simulink model "Projeto_Distribuicao"  (R2018b)
settings: Solver=VariableStepDiscrete  StartTime=0.0  StopTime=2  RelTol=1e-3
libraries: powerlib x50, powerlib_meascontrol x3
settings Model: Creator=ricar  LastModifiedBy=ricar

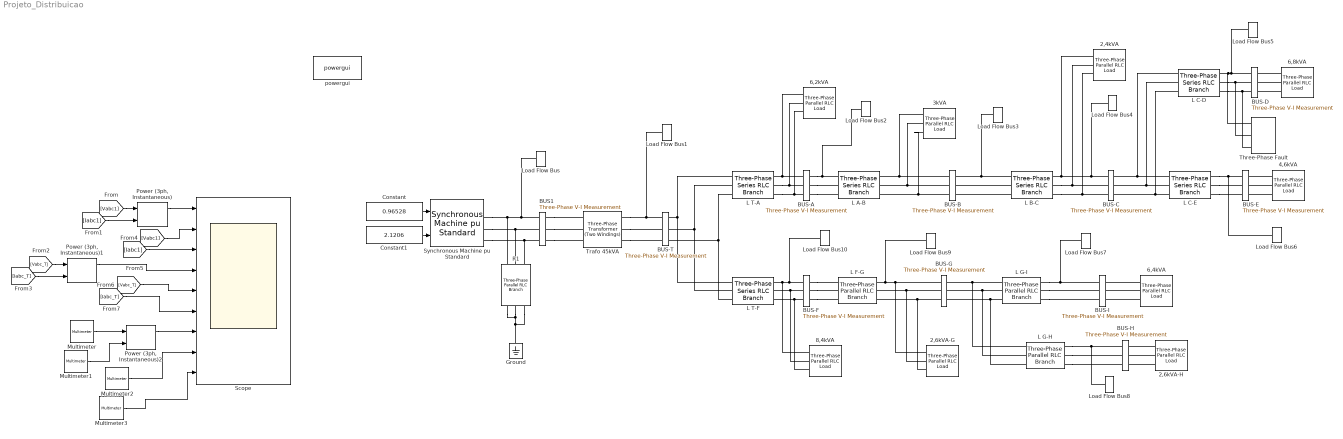
== system Projeto_Distribuicao ==
  2,4kVA : powerlib/Elements/Three-Phase Parallel RLC Load  LConnTagsString=A|B|C  Configuration=Y (grounded)  NominalVoltage=380  Vabc=[1e3 1e3 1e3]  Vabcp=[1e3 1e3 1e3]  NominalFrequency=60  UnbalancedPower=off  ActivePower=2.4e3  InductivePower=0  CapacitivePower=0  Pabc=[10e3 9e3 11e3]  QLabc=[100 90 110]  QCabc=[100 90 110]  Pabcp=[10e3 9e3 11e3]  QLabcp=[100 90 110]  QCabcp=[100 90 110]  Measurements=Branch voltages and currents  LoadType=constant Z
  2,6kVA-G : powerlib/Elements/Three-Phase Parallel RLC Load  LConnTagsString=A|B|C  Configuration=Y (grounded)  NominalVoltage=380  Vabc=[1e3 1e3 1e3]  Vabcp=[1e3 1e3 1e3]  NominalFrequency=60  UnbalancedPower=off  ActivePower=2.6e3  InductivePower=0  CapacitivePower=0  Pabc=[10e3 9e3 11e3]  QLabc=[100 90 110]  QCabc=[100 90 110]  Pabcp=[10e3 9e3 11e3]  QLabcp=[100 90 110]  QCabcp=[100 90 110]  Measurements=Branch voltages and currents  LoadType=constant Z
  2,6kVA-H : powerlib/Elements/Three-Phase Parallel RLC Load  LConnTagsString=A|B|C  Configuration=Y (grounded)  NominalVoltage=380  Vabc=[1e3 1e3 1e3]  Vabcp=[1e3 1e3 1e3]  NominalFrequency=60  UnbalancedPower=off  ActivePower=2.6e3  InductivePower=0  CapacitivePower=0  Pabc=[10e3 9e3 11e3]  QLabc=[100 90 110]  QCabc=[100 90 110]  Pabcp=[10e3 9e3 11e3]  QLabcp=[100 90 110]  QCabcp=[100 90 110]  Measurements=Branch voltages and currents  LoadType=constant Z
  3kVA : powerlib/Elements/Three-Phase Parallel RLC Load  LConnTagsString=A|B|C  Configuration=Y (grounded)  NominalVoltage=380  Vabc=[1e3 1e3 1e3]  Vabcp=[1e3 1e3 1e3]  NominalFrequency=60  UnbalancedPower=off  ActivePower=3e3  InductivePower=0  CapacitivePower=0  Pabc=[10e3 9e3 11e3]  QLabc=[100 90 110]  QCabc=[100 90 110]  Pabcp=[10e3 9e3 11e3]  QLabcp=[100 90 110]  QCabcp=[100 90 110]  Measurements=Branch voltages and currents  LoadType=constant Z
  4,6kVA : powerlib/Elements/Three-Phase Parallel RLC Load  LConnTagsString=A|B|C  Configuration=Y (grounded)  NominalVoltage=380  Vabc=[1e3 1e3 1e3]  Vabcp=[1e3 1e3 1e3]  NominalFrequency=60  UnbalancedPower=off  ActivePower=4.6e3  InductivePower=0  CapacitivePower=0  Pabc=[10e3 9e3 11e3]  QLabc=[100 90 110]  QCabc=[100 90 110]  Pabcp=[10e3 9e3 11e3]  QLabcp=[100 90 110]  QCabcp=[100 90 110]  Measurements=Branch voltages and currents  LoadType=constant Z
  6,2kVA : powerlib/Elements/Three-Phase Parallel RLC Load  LConnTagsString=A|B|C  Configuration=Y (grounded)  NominalVoltage=380  Vabc=[1e3 1e3 1e3]  Vabcp=[1e3 1e3 1e3]  NominalFrequency=60  UnbalancedPower=off  ActivePower=6.2e3  InductivePower=0  CapacitivePower=0  Pabc=[10e3 9e3 11e3]  QLabc=[100 90 110]  QCabc=[100 90 110]  Pabcp=[10e3 9e3 11e3]  QLabcp=[100 90 110]  QCabcp=[100 90 110]  Measurements=Branch voltages and currents  LoadType=constant Z
  6,4kVA : powerlib/Elements/Three-Phase Parallel RLC Load  LConnTagsString=A|B|C  Configuration=Y (grounded)  NominalVoltage=380  Vabc=[1e3 1e3 1e3]  Vabcp=[1e3 1e3 1e3]  NominalFrequency=60  UnbalancedPower=off  ActivePower=6.4e3  InductivePower=0  CapacitivePower=0  Pabc=[10e3 9e3 11e3]  QLabc=[100 90 110]  QCabc=[100 90 110]  Pabcp=[10e3 9e3 11e3]  QLabcp=[100 90 110]  QCabcp=[100 90 110]  Measurements=Branch voltages and currents  LoadType=constant Z
  6,8kVA : powerlib/Elements/Three-Phase Parallel RLC Load  LConnTagsString=A|B|C  Configuration=Y (grounded)  NominalVoltage=380  Vabc=[1e3 1e3 1e3]  Vabcp=[1e3 1e3 1e3]  NominalFrequency=60  UnbalancedPower=off  ActivePower=6.8e3  InductivePower=0  CapacitivePower=0  Pabc=[10e3 9e3 11e3]  QLabc=[100 90 110]  QCabc=[100 90 110]  Pabcp=[10e3 9e3 11e3]  QLabcp=[100 90 110]  QCabcp=[100 90 110]  Measurements=Branch voltages and currents  LoadType=constant Z
  8,4kVA : powerlib/Elements/Three-Phase Parallel RLC Load  LConnTagsString=A|B|C  Configuration=Y (grounded)  NominalVoltage=380  Vabc=[1e3 1e3 1e3]  Vabcp=[1e3 1e3 1e3]  NominalFrequency=60  UnbalancedPower=off  ActivePower=8.4e3  InductivePower=0  CapacitivePower=0  Pabc=[10e3 9e3 11e3]  QLabc=[100 90 110]  QCabc=[100 90 110]  Pabcp=[10e3 9e3 11e3]  QLabcp=[100 90 110]  QCabcp=[100 90 110]  Measurements=Branch voltages and currents  LoadType=constant Z
  BUS-A : powerlib/Measurements/Three-Phase V-I Measurement  VoltageMeasurement=phase-to-ground  SetLabelV=on  LabelV=Vabc_A  Vpu=off  VpuLL=off  CurrentMeasurement=yes  SetLabelI=on  LabelI=Iabc_A  Ipu=off  Pbase=100e6  Vbase=500e3  OutputType=Complex  PhasorSimulation=off  PSBequivalent=0
  BUS-B : powerlib/Measurements/Three-Phase V-I Measurement  VoltageMeasurement=phase-to-ground  SetLabelV=on  LabelV=Vabc_B  Vpu=off  VpuLL=off  CurrentMeasurement=yes  SetLabelI=on  LabelI=Iabc_B  Ipu=off  Pbase=100e6  Vbase=500e3  OutputType=Complex  PhasorSimulation=off  PSBequivalent=0
  BUS-C : powerlib/Measurements/Three-Phase V-I Measurement  VoltageMeasurement=phase-to-ground  SetLabelV=on  LabelV=Vabc_C  Vpu=off  VpuLL=off  CurrentMeasurement=yes  SetLabelI=on  LabelI=Iabc_C  Ipu=off  Pbase=100e6  Vbase=500e3  OutputType=Complex  PhasorSimulation=off  PSBequivalent=0
  BUS-D : powerlib/Measurements/Three-Phase V-I Measurement  VoltageMeasurement=phase-to-ground  SetLabelV=on  LabelV=Vabc_D  Vpu=off  VpuLL=off  CurrentMeasurement=yes  SetLabelI=on  LabelI=Iabc_D  Ipu=off  Pbase=100e6  Vbase=500e3  OutputType=Complex  PhasorSimulation=off  PSBequivalent=0
  BUS-E : powerlib/Measurements/Three-Phase V-I Measurement  VoltageMeasurement=phase-to-ground  SetLabelV=on  LabelV=Vabc_E  Vpu=off  VpuLL=off  CurrentMeasurement=yes  SetLabelI=on  LabelI=Iabc_E  Ipu=off  Pbase=100e6  Vbase=500e3  OutputType=Complex  PhasorSimulation=off  PSBequivalent=0
  BUS-F : powerlib/Measurements/Three-Phase V-I Measurement  VoltageMeasurement=phase-to-ground  SetLabelV=on  LabelV=Vabc_F  Vpu=off  VpuLL=off  CurrentMeasurement=yes  SetLabelI=on  LabelI=Iabc_F  Ipu=off  Pbase=100e6  Vbase=500e3  OutputType=Complex  PhasorSimulation=off  PSBequivalent=0
  BUS-G : powerlib/Measurements/Three-Phase V-I Measurement  VoltageMeasurement=phase-to-ground  SetLabelV=on  LabelV=Vabc_G  Vpu=off  VpuLL=off  CurrentMeasurement=yes  SetLabelI=on  LabelI=Iabc_G  Ipu=off  Pbase=100e6  Vbase=500e3  OutputType=Complex  PhasorSimulation=off  PSBequivalent=0
  BUS-H : powerlib/Measurements/Three-Phase V-I Measurement  VoltageMeasurement=phase-to-ground  SetLabelV=on  LabelV=Vabc_H  Vpu=off  VpuLL=off  CurrentMeasurement=yes  SetLabelI=on  LabelI=Iabc_H  Ipu=off  Pbase=100e6  Vbase=500e3  OutputType=Complex  PhasorSimulation=off  PSBequivalent=0
  BUS-I : powerlib/Measurements/Three-Phase V-I Measurement  VoltageMeasurement=phase-to-ground  SetLabelV=on  LabelV=Vabc_I  Vpu=off  VpuLL=off  CurrentMeasurement=yes  SetLabelI=on  LabelI=Iabc_I  Ipu=off  Pbase=100e6  Vbase=500e3  OutputType=Complex  PhasorSimulation=off  PSBequivalent=0
  BUS-T : powerlib/Measurements/Three-Phase V-I Measurement  VoltageMeasurement=phase-to-ground  SetLabelV=on  LabelV=Vabc_T  Vpu=off  VpuLL=off  CurrentMeasurement=yes  SetLabelI=on  LabelI=Iabc_T  Ipu=off  Pbase=100e6  Vbase=500e3  OutputType=Complex  PhasorSimulation=off  PSBequivalent=0
  BUS1 : powerlib/Measurements/Three-Phase V-I Measurement  VoltageMeasurement=phase-to-ground  SetLabelV=on  LabelV=Vabc1  Vpu=off  VpuLL=off  CurrentMeasurement=yes  SetLabelI=on  LabelI=Iabc1  Ipu=off  Pbase=100e6  Vbase=500e3  OutputType=Complex  PhasorSimulation=off  PSBequivalent=0
  Constant : Constant  Value=0.96528
  Constant1 : Constant  Value=2.1206
  Ground : powerlib/Elements/Ground  LConnTagsString=a
  L A-B : powerlib/Elements/Three-Phase Series RLC Branch  LConnTagsString=A|B|C  RConnTagsString=A|B|C  BranchType=R  Resistance=0.032585  Inductance=1e-3  Capacitance=1e-6  Measurements=None
  L B-C : powerlib/Elements/Three-Phase Series RLC Branch  LConnTagsString=A|B|C  RConnTagsString=A|B|C  BranchType=R  Resistance=0.0300125  Inductance=1e-3  Capacitance=1e-6  Measurements=None
  L C-D : powerlib/Elements/Three-Phase Series RLC Branch  LConnTagsString=A|B|C  RConnTagsString=A|B|C  BranchType=R  Resistance=0.0343  Inductance=1e-3  Capacitance=1e-6  Measurements=None
  L C-E : powerlib/Elements/Three-Phase Series RLC Branch  LConnTagsString=A|B|C  RConnTagsString=A|B|C  BranchType=R  Resistance=0.0343  Inductance=1e-3  Capacitance=1e-6  Measurements=None
  L F-G : powerlib/Elements/Three-Phase Parallel RLC Branch  LConnTagsString=A|B|C  RConnTagsString=A|B|C  BranchType=R  Resistance=0.0188531  Inductance=0  Capacitance=0  Measurements=None
      settings: SourceProductName=Simscape Power Systems  SourceProductBaseCode=PS
  L G-H : powerlib/Elements/Three-Phase Parallel RLC Branch  LConnTagsString=A|B|C  RConnTagsString=A|B|C  BranchType=R  Resistance=0.042875  Inductance=0  Capacitance=0  Measurements=None
      settings: SourceProductName=Simscape Power Systems  SourceProductBaseCode=PS
  L G-I : powerlib/Elements/Three-Phase Parallel RLC Branch  LConnTagsString=A|B|C  RConnTagsString=A|B|C  BranchType=R  Resistance=0.0300125  Inductance=0  Capacitance=0  Measurements=None
      settings: SourceProductName=Simscape Power Systems  SourceProductBaseCode=PS
  L T-A : powerlib/Elements/Three-Phase Series RLC Branch  LConnTagsString=A|B|C  RConnTagsString=A|B|C  BranchType=R  Resistance=0.0107732  Inductance=1e-3  Capacitance=1e-6  Measurements=None
  L T-F : powerlib/Elements/Three-Phase Series RLC Branch  LConnTagsString=A|B|C  RConnTagsString=A|B|C  BranchType=R  Resistance=0.0134665  Inductance=1e-3  Capacitance=1e-6  Measurements=None
  Load Flow Bus : powerlib/Measurements/Load Flow Bus  LConnTagsString=a  Phases=single  Connectors=on one side  ID=BUS_1  Vbase=13.8e3  Vref=1  Vangle=0  VLF=1  VLFb=1  VLFc=1  angleLF=0  angleLFb=0  angleLFc=0
      settings: SourceProductName=Simscape Power Systems
  Load Flow Bus1 : powerlib/Measurements/Load Flow Bus  LConnTagsString=a  Phases=single  Connectors=on one side  ID=BUS_T  Vbase=380  Vref=1  Vangle=0  VLF=0.9848  VLFb=1  VLFc=1  angleLF=-8.624  angleLFb=0  angleLFc=0
      settings: SourceProductName=Simscape Power Systems
  Load Flow Bus10 : powerlib/Measurements/Load Flow Bus  LConnTagsString=a  Phases=single  Connectors=on one side  ID=BUS_F  Vbase=380  Vref=1  Vangle=0  VLF=0.983  VLFb=1  VLFc=1  angleLF=-8.624  angleLFb=0  angleLFc=0
      settings: SourceProductName=Simscape Power Systems
  Load Flow Bus2 : powerlib/Measurements/Load Flow Bus  LConnTagsString=a  Phases=single  Connectors=on one side  ID=BUS_A  Vbase=380  Vref=1  Vangle=0  VLF=0.9831  VLFb=1  VLFc=1  angleLF=-8.624  angleLFb=0  angleLFc=0
      settings: SourceProductName=Simscape Power Systems
  Load Flow Bus3 : powerlib/Measurements/Load Flow Bus  LConnTagsString=a  Phases=single  Connectors=on one side  ID=BUS_B  Vbase=380  Vref=1  Vangle=0  VLF=0.9794  VLFb=1  VLFc=1  angleLF=-8.624  angleLFb=0  angleLFc=0
      settings: SourceProductName=Simscape Power Systems
  Load Flow Bus4 : powerlib/Measurements/Load Flow Bus  LConnTagsString=a  Phases=single  Connectors=on one side  ID=BUS_C  Vbase=380  Vref=1  Vangle=0  VLF=0.9766  VLFb=1  VLFc=1  angleLF=-8.624  angleLFb=0  angleLFc=0
      settings: SourceProductName=Simscape Power Systems
  Load Flow Bus5 : powerlib/Measurements/Load Flow Bus  LConnTagsString=a  Phases=single  Connectors=on one side  ID=BUS_D  Vbase=380  Vref=1  Vangle=0  VLF=0.975  VLFb=1  VLFc=1  angleLF=-8.624  angleLFb=0  angleLFc=0
      settings: SourceProductName=Simscape Power Systems
  Load Flow Bus6 : powerlib/Measurements/Load Flow Bus  LConnTagsString=a  Phases=single  Connectors=on one side  ID=BUS_E  Vbase=380  Vref=1  Vangle=0  VLF=0.9756  VLFb=1  VLFc=1  angleLF=-8.624  angleLFb=0  angleLFc=0
      settings: SourceProductName=Simscape Power Systems
  Load Flow Bus7 : powerlib/Measurements/Load Flow Bus  LConnTagsString=a  Phases=single  Connectors=on one side  ID=BUS_I  Vbase=380  Vref=1  Vangle=0  VLF=0.9802  VLFb=1  VLFc=1  angleLF=-8.624  angleLFb=0  angleLFc=0
      settings: SourceProductName=Simscape Power Systems
  Load Flow Bus8 : powerlib/Measurements/Load Flow Bus  LConnTagsString=a  Phases=single  Connectors=on one side  ID=BUS_H  Vbase=380  Vref=1  Vangle=0  VLF=0.9807  VLFb=1  VLFc=1  angleLF=-8.624  angleLFb=0  angleLFc=0
      settings: SourceProductName=Simscape Power Systems
  Load Flow Bus9 : powerlib/Measurements/Load Flow Bus  LConnTagsString=a  Phases=single  Connectors=on one side  ID=BUS_G  Vbase=380  Vref=1  Vangle=0  VLF=0.9815  VLFb=1  VLFc=1  angleLF=-8.624  angleLFb=0  angleLFc=0
      settings: SourceProductName=Simscape Power Systems
  Multimeter : powerlib/Measurements/Multimeter  PhasorSimulation=off  OutputType=Complex  sel=[22 23 24]  L=54  Gain=[1 1 1]  yselected={'Uag: 6,8kVA','Ubg: 6,8kVA','Ucg: 6,8kVA'};  PSBOutputType=1  PSBequivalent=0  AxesSetting=[0,0.1,-100,100]  Display=0  SavedBlockNames=-11
  Multimeter1 : powerlib/Measurements/Multimeter  PhasorSimulation=off  OutputType=Complex  sel=[49 50 51]  L=54  Gain=[1 1 1]  yselected={'Iag: 6,8kVA','Ibg: 6,8kVA','Icg: 6,8kVA'};  PSBOutputType=1  PSBequivalent=0  AxesSetting=[0,0.1,-100,100]  Display=0  SavedBlockNames=-11
  Multimeter2 : powerlib/Measurements/Multimeter  PhasorSimulation=off  OutputType=Complex  sel=[22 23 24]  L=54  Gain=[1 1 1]  yselected={'Uag: 6,8kVA','Ubg: 6,8kVA','Ucg: 6,8kVA'};  PSBOutputType=1  PSBequivalent=0  AxesSetting=[0,0.1,-100,100]  Display=0  SavedBlockNames=-11
  Multimeter3 : powerlib/Measurements/Multimeter  PhasorSimulation=off  OutputType=Complex  sel=[49 50 51]  L=54  Gain=[1 1 1]  yselected={'Iag: 6,8kVA','Ibg: 6,8kVA','Icg: 6,8kVA'};  PSBOutputType=1  PSBequivalent=0  AxesSetting=[0,0.1,-100,100]  Display=0  SavedBlockNames=-11
  "Power (3ph, Instantaneous)" : powerlib_meascontrol/Measurements/Power (3ph, Instantaneous)
      settings: SourceProductName=Simscape Power Systems
  "Power (3ph, Instantaneous)1" : powerlib_meascontrol/Measurements/Power (3ph, Instantaneous)
      settings: SourceProductName=Simscape Power Systems
  "Power (3ph, Instantaneous)2" : powerlib_meascontrol/Measurements/Power (3ph, Instantaneous)
      settings: SourceProductName=Simscape Power Systems
  R1 : powerlib/Elements/Three-Phase Parallel RLC Branch  LConnTagsString=A|B|C  RConnTagsString=A|B|C  BranchType=R  Resistance=1e+6  Inductance=1e-3  Capacitance=1e-6  Measurements=None
      settings: SourceProductName=Simscape Power Systems  SourceProductBaseCode=PS
  Scope : Scope  NumInputPorts=9
  Synchronous Machine pu Standard : powerlib/Machines/Synchronous Machine pu Standard  PresetModel=No  MechanicalLoad=Mechanical power Pm  ShowDetailedParameters=on  RotorType=Round  Units=per unit standard parameters  MeasurementBus=off  NominalParameters=[45e+03 13800 60]  Reactances1=[ 1.81, 0.3, 0.23, 1.76, 0.65, 0.25, 0.15 ]  Reactances2=[2.24 0.17 0.12 1.02 0.13 0.08]  dAxisTimeConstants=Short-circuit  qAxisTimeConstants=Short-circuit  TimeConstants1="[ 4.4849  0.0681  0.1  ]"  TimeConstants2=[ 8.0, 0.03, 1.0, 0.07 ]  TimeConstants3="[  4.49  0.0681  0.0513  ]"  TimeConstants4=[ 8.0, 0.03, 0.3371, 0.0295 ]  TimeConstants5=[ 1.01, 0.053, 0.1 ]  TimeConstants6=[ 1.3201, 0.023, 1.0, 0.07 ]  TimeConstants7=[0.012 0.003 0.003]  TimeConstants8=[ 1.3201, 0.0231, 0.3371, 0.0295 ]  StatorResistance=0.037875  Mechanical=[0.1028 0.02056 2]  PolePairs=20  InitialConditions=[0 -38.2008 0.942468 0.942468 0.942468 -8.69634 -128.696 111.304 2.12064]  SetSaturation=off  Saturation=[0.6404,0.7127,0.8441,0.9214,0.9956,1.082,1.19,1.316,1.457;0.7,0.7698,0.8872,0.9466,0.9969,1.046,1.1,1.151,1.201]  LoadFlowParameters=[1,0,0,0,0]  TsPowergui=0  TsBlock=-1  IterativeModel=Trapezoidal non iterative  IterativeDiscreteModel=Trapezoidal non iterative  BusType=swing  Pref=0  Qref=0  Qmin=-inf  Qmax=inf  PLF=0  QLF=0
      settings: SourceProductName=Simscape Power Systems
  Three-Phase Fault : powerlib/Elements/Three-Phase Fault  InitialStates=0  FaultA=on  FaultB=off  FaultC=off  GroundFault=on  SwitchTimes="[0.2  0.5]"  External=off  SwitchStatus=NaN  FaultResistance=0.001  GroundResistance=0.01  SnubberResistance=1e6  SnubberCapacitance=inf  Measurements=None
  Trafo 45kVA : powerlib/Elements/Three-Phase Transformer (Two Windings)  Winding1Connection=Yg  Winding2Connection=Yg  CoreType=Three single-phase transformers  SetSaturation=off  Hysteresis=off  DataFile='hysteresis'  SetInitialFlux=off  Measurements=None  UNITS=pu  NominalPower=[ 45e3 , 60 ]  Winding1=[ 13.8e3 , 0.002 , 0.08 ]  Winding2=[ 380 , 0.002 , 0.08 ]  Rm=500  Lm=500  L0=0.5  Saturation=[ 0,0 ; 0.0024,1.2 ; 1.0,1.52 ]  InitialFluxes=[ 0.8 , -0.8 , 0.7 ]  MoreParameters=off  BreakLoop=off  DataType=off  TransfoNumber=1
  powergui : powerlib/powergui  Priority=1  SimulationMode=Discrete  SampleTime=50e-6  frequency=60  Iterations=1000  frequencyindice=60  Pbase=100e3  ErrMax=0.0001  UnitsV=V  UnitsW=kW  buscounter=0  FunctionMessages=off  echomessages=off  EnableUseOfTLC=off  CurrentSourceSwitches=off  DisableSnubberDevices=off  DisableRonSwitches=off  DisableVfSwitches=off  DisplayEquations=off  SolverType=Tustin/Backward Euler (TBE)  Interpol=off  ExternalGateDelay=off  methode=off  Ts=100  x0status=blocks  SPID=on  SwTol=0  HookPort=off  RestoreLinks=warning  ResistiveCurrentMeasurement=off  Frange=[0:2:500]  Ylog=off  Xlog=on  ShowGrid=off  save=off  variable=ZData  structure=0  ZoomFFT=off  StartTime=0.0  cycles=1  DisplayStyle=1  fundamental=60  FreqAxis=off  MaxFrequency=1000  frequencyindicesteady=1  RmsSteady=1  display=off
  wires:
  Constant/1 -> Synchronous Machine pu Standard/1
  Constant1/1 -> Synchronous Machine pu Standard/2
  [Iabc1] -> "Power (3ph, Instantaneous)"/2
  [Vabc1] -> "Power (3ph, Instantaneous)"/1
  "Power (3ph, Instantaneous)"/1 -> Scope/1
  [Iabc_T] -> "Power (3ph, Instantaneous)1"/2
  [Vabc_T] -> "Power (3ph, Instantaneous)1"/1
  Multimeter/1 -> "Power (3ph, Instantaneous)2"/1
  Multimeter1/1 -> "Power (3ph, Instantaneous)2"/2
  "Power (3ph, Instantaneous)1"/1 -> Scope/4
  "Power (3ph, Instantaneous)2"/1 -> Scope/7
  [Vabc1] -> Scope/2
  [Iabc1] -> Scope/3
  [Vabc_T] -> Scope/5
  [Iabc_T] -> Scope/6
  Multimeter2/1 -> Scope/8
  Multimeter3/1 -> Scope/9
  connections:
  R1/LConn1 -- Synchronous Machine pu Standard/RConn1 -- Load Flow Bus/LConn1 -- BUS1/LConn1
  R1/LConn2 -- Synchronous Machine pu Standard/RConn2 -- BUS1/LConn2
  R1/LConn3 -- Synchronous Machine pu Standard/RConn3 -- BUS1/LConn3
  BUS1/RConn1 -- Trafo 45kVA/LConn1
  BUS1/RConn2 -- Trafo 45kVA/LConn2
  BUS1/RConn3 -- Trafo 45kVA/LConn3
  Trafo 45kVA/RConn1 -- Load Flow Bus1/LConn1 -- BUS-T/LConn1
  Trafo 45kVA/RConn2 -- BUS-T/LConn2
  Trafo 45kVA/RConn3 -- BUS-T/LConn3
  BUS-T/RConn1 -- L T-F/LConn1 -- L T-A/LConn1
  BUS-T/RConn2 -- L T-F/LConn2 -- L T-A/LConn2
  BUS-T/RConn3 -- L T-F/LConn3 -- L T-A/LConn3
  L T-A/RConn1 -- 6,2kVA/LConn1 -- BUS-A/LConn1
  L T-A/RConn2 -- 6,2kVA/LConn2 -- BUS-A/LConn2
  L T-A/RConn3 -- 6,2kVA/LConn3 -- BUS-A/LConn3
  BUS-A/RConn1 -- Load Flow Bus2/LConn1 -- L A-B/LConn1
  BUS-A/RConn2 -- L A-B/LConn2
  BUS-A/RConn3 -- L A-B/LConn3
  L T-F/RConn1 -- 8,4kVA/LConn1 -- Load Flow Bus10/LConn1 -- BUS-F/LConn1
  L T-F/RConn2 -- 8,4kVA/LConn2 -- BUS-F/LConn2
  L T-F/RConn3 -- 8,4kVA/LConn3 -- BUS-F/LConn3
  BUS-F/RConn1 -- L F-G/LConn1
  BUS-F/RConn2 -- L F-G/LConn2
  BUS-F/RConn3 -- L F-G/LConn3
  BUS-B/LConn1 -- 3kVA/LConn1 -- L A-B/RConn1
  BUS-B/LConn2 -- 3kVA/LConn2 -- L A-B/RConn2
  BUS-B/LConn3 -- 3kVA/LConn3 -- L A-B/RConn3
  BUS-G/LConn1 -- 2,6kVA-G/LConn1 -- Load Flow Bus9/LConn1 -- L F-G/RConn1
  BUS-G/LConn2 -- 2,6kVA-G/LConn2 -- L F-G/RConn2
  BUS-G/LConn3 -- 2,6kVA-G/LConn3 -- L F-G/RConn3
  L B-C/LConn3 -- BUS-B/RConn3
  L B-C/LConn2 -- BUS-B/RConn2
  L B-C/LConn1 -- Load Flow Bus3/LConn1 -- BUS-B/RConn1
  L G-I/RConn1 -- Load Flow Bus7/LConn1 -- BUS-I/LConn1
  L G-I/RConn2 -- BUS-I/LConn2
  L G-I/RConn3 -- BUS-I/LConn3
  L G-H/RConn1 -- Load Flow Bus8/LConn1 -- BUS-H/LConn1
  L G-H/RConn2 -- BUS-H/LConn2
  L G-H/RConn3 -- BUS-H/LConn3
  L B-C/RConn1 -- 2,4kVA/LConn1 -- Load Flow Bus4/LConn1 -- BUS-C/LConn1
  L B-C/RConn2 -- 2,4kVA/LConn2 -- BUS-C/LConn2
  L B-C/RConn3 -- 2,4kVA/LConn3 -- BUS-C/LConn3
  L C-D/RConn1 -- Three-Phase Fault/LConn1 -- Load Flow Bus5/LConn1 -- BUS-D/LConn1
  L C-D/RConn2 -- Three-Phase Fault/LConn2 -- BUS-D/LConn2
  L C-D/RConn3 -- Three-Phase Fault/LConn3 -- BUS-D/LConn3
  L C-E/RConn1 -- Load Flow Bus6/LConn1 -- BUS-E/LConn1
  L C-E/RConn2 -- BUS-E/LConn2
  L C-E/RConn3 -- BUS-E/LConn3
  6,4kVA/LConn1 -- BUS-I/RConn1
  6,4kVA/LConn2 -- BUS-I/RConn2
  6,4kVA/LConn3 -- BUS-I/RConn3
  2,6kVA-H/LConn1 -- BUS-H/RConn1
  2,6kVA-H/LConn2 -- BUS-H/RConn2
  2,6kVA-H/LConn3 -- BUS-H/RConn3
  4,6kVA/LConn1 -- BUS-E/RConn1
  4,6kVA/LConn2 -- BUS-E/RConn2
  4,6kVA/LConn3 -- BUS-E/RConn3
  6,8kVA/LConn1 -- BUS-D/RConn1
  6,8kVA/LConn2 -- BUS-D/RConn2
  6,8kVA/LConn3 -- BUS-D/RConn3
  L G-I/LConn1 -- L G-H/LConn1 -- BUS-G/RConn1
  L G-I/LConn2 -- L G-H/LConn2 -- BUS-G/RConn2
  L G-I/LConn3 -- L G-H/LConn3 -- BUS-G/RConn3
  L C-E/LConn1 -- L C-D/LConn1 -- BUS-C/RConn1
  L C-E/LConn2 -- L C-D/LConn2 -- BUS-C/RConn2
  L C-E/LConn3 -- L C-D/LConn3 -- BUS-C/RConn3
  R1/RConn1 -- R1/RConn2 -- R1/RConn3 -- Ground/LConn1
